simulink model "flexpwm_ctu_etimer"  (Simulink 8.1)
settings: Solver=FixedStepDiscrete  StartTime=0.0  StopTime=10.0  FixedStep=0.2  RelTol=1e-3
undefined symbols (not defined in the file or in its folder): A14, A15, B, B13, B7, D, L3, P3, PC10, PC14, PD4, PD6, R10
libraries: rappid_564xl_ec_toolbox x9
settings Model: Creator=evarshavskaya  LastModifiedBy=evarshavskaya
settings DataIOCC: ExternalInput=off  InitialState=off  SaveOutput=off  SignalLogging=off  SaveTime=off
settings OptimizationCC: InlineParams=on  OptimizeModelRefInitCode=on  LifeSpan=1
settings DebuggingCC: InheritedTsInSrcMsg=none  SingleTaskRateTransMsg=error  UnconnectedInputMsg=error  UnconnectedOutputMsg=error  UnconnectedLineMsg=error  UnknownTsInhSupMsg=error
settings HardwareCC: ProdLargestAtomicInteger=Long  ProdLargestAtomicFloat=Double  ProdIntDivRoundTo=Zero  ProdEndianess=BigEndian  ProdHWDeviceType=Freescale->32-bit PowerPC
settings RTWCC: SystemTargetFile=rappid564xl.tlc  MakeCommand=rappid_564xl_make_rtw  TemplateMakefile=rappid_564xl_default_tmf  PostCodeGenCommand=rappid_analyzegencode(buildInfo)  Description=RAppID Toolbox MPC564xL Code Generation Target (rappid)  ProcessScript=rappid564xl_make_rtw_hook
settings CodeAppCC: IgnoreCustomStorageClasses=off  CustomSymbolStrType=$N$R$M  InternalIdentifier=Classic
settings STFCustomTargetCC: CodeReplacementLibrary=ANSI_C  ModelReferenceCompliant=off  CombineOutputUpdateFcns=on  SuppressErrorStatus=on  ERTCustomFileBanners=on  SupportContinuousTime=off  SupportNonInlinedSFcns=off  MATLABClassNameForMDSCustomization=Simulink.SoftwareTarget.ERTCustomization  GRTInterface=off  SystemTargetFile=rappid564xl.tlc
settings ERTTargetCC: CodeReplacementLibrary=ANSI_C  MultiwordLength=2048  ModelReferenceCompliant=off  ParMdlRefBuildCompliant=off  CompOptLevelCompliant=off  ConcurrentExecutionCompliant=off  SuppressErrorStatus=on  ERTFirstTimeCompliant=off  ModelStepFunctionPrototypeControlCompliant=off  CPPClassGenCompliant=off  ExtModeMexFile=noextcomm  InlinedParameterPlacement=NonHierarchical  ERTCustomFileTemplate=example_file_process.tlc  ConvertIfToSwitch=off  SuppressUnreachableDefaultCases=off

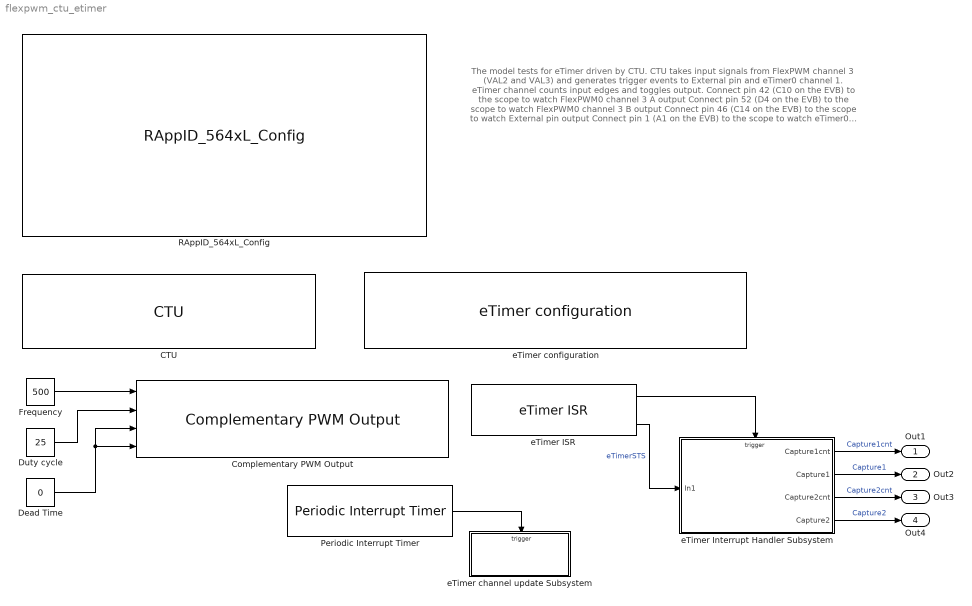
== system flexpwm_ctu_etimer ==
  note: The model tests for eTimer driven by CTU.
      |
      | CTU takes input signals from FlexPWM channel 3 (VAL2 and VAL3) and generates trigger events
      | to External pin and eTimer0 channel 1. eTimer channel counts input edges and toggles output.
      |
      | Connect pin 42 (C10 on the EVB) to the scope to watch FlexPWM0 channel 3 A output
      | Connect pin 52 (D4 on the EVB) to the scope to watch FlexPWM0 channel 3 B output
      | Connect pin 46 (C14 on the EVB) to the scope to watch External pin output
      | Connect pin 1  (A1 on the EVB) to the scope to watch eTimer0 channel 1 output
      | Connect pin 54 (D6 on the EVB) to the scope to watch eTimer0 channel 1 interrupt
  CTU : rappid_564xl_ec_toolbox/MPC564xL/Motor Control Blocks/CTU  ModeEdit=Triggered  Mode=0  MRSedit=PWM reload Rising edge  MRS=0  MaxDelay=1000  ExtTgrPin_0="46  : PC14 : [ 103 ] : [ E15 ]"  ExtInPin_0=None  extTgrPcr=46  extInPcr=255  InputSelection=16843008  PWM_REL=Disabled  PWM_ODD_0=Disabled  PWM_ODD_1=Disabled  PWM_ODD_2=Disabled  PWM_ODD_3=Rising  PWM_EVEN_0=Disabled  PWM_EVEN_1=Disabled  PWM_EVEN_2=Disabled  PWM_EVEN_3=Rising  RPWM_0=Disabled  RPWM_1=Disabled  RPWM_2=Disabled  RPWM_3=Rising  eTimer_0=Disabled  eTimer_1=Disabled  External=Disabled  TriggerOutput_1=98  TriggerOutput_2=0  ADC_CmdIndex_1=0  ADC_CmdIndex_2=0  ADC_Cmd_1=16384  ADC_Cmd_2=0  ADC_Cmd_3=0  ADC_Cmd_4=0  ADC_Cmd_5=0  ADC_Cmd_6=0  ADC_Cmd_7=0  ADC_Cmd_8=0  ADC_Cmd_9=0  ADC_Cmd_10=0  ADC_Cmd_11=0  ADC_Cmd_12=0  ADC_Cmd_13=0  ADC_Cmd_14=0  ADC_Cmd_15=0  ADC_Cmd_16=0  ADC_Cmd_17=0  ADC_Cmd_18=0  ADC_Cmd_19=0  ADC_Cmd_20=0  ADC_Cmd_21=0  ADC_Cmd_22=0  ADC_Cmd_23=0  ADC_Cmd_24=0  T0_E=on  T0_ETE=on  T0_T0E=on  T0_T1E=off  T0_T2E=off  T0_ADCE=off  T0_Delay=250  T1_E=off  T1_ETE=off  T1_T0E=off  T1_T1E=off  T1_T2E=off  T1_ADCE=off  T1_Delay=250  T2_E=off  T2_ETE=off  T2_T0E=off  T2_T1E=off  T2_T2E=off  T2_ADCE=off  T2_Delay=0  T3_E=off  T3_ETE=off  T3_T0E=off  T3_T1E=off  T3_T2E=off  T3_ADCE=off  T3_Delay=0  T4_E=off  T4_ETE=off  T4_T0E=off  T4_T1E=off  T4_T2E=off  T4_ADCE=off  T4_Delay=0  T5_E=off  T5_ETE=off  T5_T0E=off  T5_T1E=off  T5_T2E=off  T5_ADCE=off  T5_Delay=0  T6_E=off  T6_ETE=off  T6_T0E=off  T6_T1E=off  T6_T2E=off  T6_ADCE=off  T6_Delay=0  T7_E=off  T7_ETE=off  T7_T0E=off  T7_T1E=off  T7_T2E=off  T7_ADCE=off  T7_Delay=0  T_delay=0  ADC_Cmd=0  T0_ADC_num=0  T0_ADC_nlist=no commands  T1_ADC_num=0  T1_ADC_nlist=no commands  T2_ADC_num=0  T2_ADC_nlist=no commands  T3_ADC_num=0  T3_ADC_nlist=no commands  T4_ADC_num=0  T4_ADC_nlist=no commands  T5_ADC_num=0  T5_ADC_nlist=no commands  T6_ADC_num=0  T6_ADC_nlist=no commands  T7_ADC_num=0  T7_ADC_nlist=no commands  ADC_CMS_1=Single-conversion mode: ADC unit A  ADC_CIR_1=Disabled  ADC_FIFO_1=0  ADC_CHA_1=0  ADC_CHB_1=0  ADC_CMS_2=Single-conversion mode: ADC unit A  ADC_CIR_2=Disabled  ADC_FIFO_2=0  ADC_CHA_2=0  ADC_CHB_2=0  ADC_CMS_3=Single-conversion mode: ADC unit A  ADC_CIR_3=Disabled  ADC_FIFO_3=0  ADC_CHA_3=0  ADC_CHB_3=0  ADC_CMS_4=Single-conversion mode: ADC unit A  ADC_CIR_4=Disabled  ADC_FIFO_4=0  ADC_CHA_4=0  ADC_CHB_4=0  ADC_CMS_5=Single-conversion mode: ADC unit A  ADC_CIR_5=Disabled  ADC_FIFO_5=0  ADC_CHA_5=0  ADC_CHB_5=0  ADC_CMS_6=Single-conversion mode: ADC unit A  ADC_CIR_6=Disabled  ADC_FIFO_6=0  ADC_CHA_6=0  ADC_CHB_6=0  ADC_CMS_7=Single-conversion mode: ADC unit A  ADC_CIR_7=Disabled  ADC_FIFO_7=0  ADC_CHA_7=0  ADC_CHB_7=0  ADC_CMS_8=Single-conversion mode: ADC unit A  ADC_CIR_8=Disabled  ADC_FIFO_8=0  ADC_CHA_8=0  ADC_CHB_8=0  ADC_CMS_9=Single-conversion mode: ADC unit A  ADC_CIR_9=Disabled  ADC_FIFO_9=0  ADC_CHA_9=0  ADC_CHB_9=0  ADC_CMS_10=Single-conversion mode: ADC unit A  ADC_CIR_10=Disabled  ADC_FIFO_10=0  ADC_CHA_10=0  ADC_CHB_10=0  ADC_CMS_11=Single-conversion mode: ADC unit A  ADC_CIR_11=Disabled  ADC_FIFO_11=0  ADC_CHA_11=0  ADC_CHB_11=0  ADC_CMS_12=Single-conversion mode: ADC unit A  ADC_CIR_12=Disabled  ADC_FIFO_12=0  ADC_CHA_12=0  ADC_CHB_12=0  ADC_CMS_13=Single-conversion mode: ADC unit A  ADC_CIR_13=Disabled  ADC_FIFO_13=0  ADC_CHA_13=0  ADC_CHB_13=0  ADC_CMS_14=Single-conversion mode: ADC unit A  ADC_CIR_14=Disabled  ADC_FIFO_14=0  ADC_CHA_14=0  ADC_CHB_14=0  ADC_CMS_15=Single-conversion mode: ADC unit A  ADC_CIR_15=Disabled  ADC_FIFO_15=0  ADC_CHA_15=0  ADC_CHB_15=0  ADC_CMS_16=Single-conversion mode: ADC unit A  ADC_CIR_16=Disabled  ADC_FIFO_16=0  ADC_CHA_16=0  ADC_CHB_16=0  ADC_CMS_17=Single-conversion mode: ADC unit A  ADC_CIR_17=Disabled  ADC_FIFO_17=0  ADC_CHA_17=0  ADC_CHB_17=0  ADC_CMS_18=Single-conversion mode: ADC unit A  ADC_CIR_18=Disabled  ADC_FIFO_18=0  ADC_CHA_18=0  ADC_CHB_18=0  ADC_CMS_19=Single-conversion mode: ADC unit A  ADC_CIR_19=Disabled  ADC_FIFO_19=0  ADC_CHA_19=0  ADC_CHB_19=0  ADC_CMS_20=Single-conversion mode: ADC unit A  ADC_CIR_20=Disabled  ADC_FIFO_20=0  ADC_CHA_20=0  ADC_CHB_20=0  ADC_CMS_21=Single-conversion mode: ADC unit A  ADC_CIR_21=Disabled  ADC_FIFO_21=0  ADC_CHA_21=0  ADC_CHB_21=0  ADC_CMS_22=Single-conversion mode: ADC unit A  ADC_CIR_22=Disabled  ADC_FIFO_22=0  ADC_CHA_22=0  ADC_CHB_22=0  ADC_CMS_23=Single-conversion mode: ADC unit A  ADC_CIR_23=Disabled  ADC_FIFO_23=0  ADC_CHA_23=0  ADC_CHB_23=0  ADC_CMS_24=Single-conversion mode: ADC unit A  ADC_CIR_24=Disabled  ADC_FIFO_24=0  ADC_CHA_24=0  ADC_CHB_24=0  dst=|  T0_cmdNum=1  T0_ADC_CMS_1=Single-conversion mode: ADC unit A  T0_ADC_CIR_1=Disabled  T0_ADC_FIFO_1=0  T0_ADC_CHA_1=0  T0_ADC_CHB_1=0  T0_ADC_CMS_2=Single-conversion mode: ADC unit A  T0_ADC_CIR_2=Disabled  T0_ADC_FIFO_2=0  T0_ADC_CHA_2=0  T0_ADC_CHB_2=0  T0_ADC_CMS_3=Single-conversion mode: ADC unit A  T0_ADC_CIR_3=Disabled  T0_ADC_FIFO_3=0  T0_ADC_CHA_3=0  T0_ADC_CHB_3=0  T1_cmdNum=1  T1_ADC_CMS_1=Single-conversion mode: ADC unit A  T1_ADC_CIR_1=Disabled  T1_ADC_FIFO_1=0  T1_ADC_CHA_1=3  T1_ADC_CHB_1=0  T1_ADC_CMS_2=Single-conversion mode: ADC unit A  T1_ADC_CIR_2=Disabled  T1_ADC_FIFO_2=0  T1_ADC_CHA_2=0  T1_ADC_CHB_2=0  T1_ADC_CMS_3=Single-conversion mode: ADC unit A  T1_ADC_CIR_3=Disabled  T1_ADC_FIFO_3=0  T1_ADC_CHA_3=0  T1_ADC_CHB_3=0  ver=2
      | Triggered mode
      |       Input selection: 00000001 00000001 00000001 00000000
      | Trigger Output 0-3: 00000000 00000000 00000000 01100010
      | Trigger Output 4-7: 00000000 00000000 00000000 00000000
      | ADC command list size: 0
  Complementary PWM Output : rappid_564xl_ec_toolbox/MPC564xL/Motor Control Blocks/Complementary PWM Output  pwmModule=0  pwmMod=0  SubModule=3  subMod=3  InitFreq=500  resolution=1 %  resValue=1  InitDuty=25  pwm45=off  pwm45en=0  InitDutyB=0  DeadTime=0  dt=IPBus clock cycles  deadtime_mks=0  debugSw=off  debug_mode=0  pin_A0=None  pin_B0=None  pin_A1=None  pin_B1=None  pin_A2=None  pin_B2=None  pin_A3="42  : PC10 : [ 111 ] : [ A15 ]"  pin_B3="52  : PD4  : [ 129 ] : [ B7 ]"  pin1_A0=None  pin1_B0=None  pin1_A1=None  pin1_B1=None  pin1_A2=None  pin1_B2=None  pin1_A3=None  pin1_B3=None  pcrNumA=42  pcrNumB=52  polA=off  polB=off  octrl=0  syncFrom0=off  masterSync=0  outVal0=off  outVal1=off  outVal2=on  outVal3=on  outVal4=on  outVal5=on  outTrig=12
  Dead Time : Constant  Value=0  OutDataTypeStr=uint32
  Duty cycle : Constant  Value=25  OutDataTypeStr=uint32
  Frequency : Constant  Value=500  OutDataTypeStr=uint32
  Periodic Interrupt Timer : rappid_564xl_ec_toolbox/MPC564xL/General Purpose Blocks/Periodic Interrupt Timer  pit_chan=1  pit_timeout=200  int_priority=13  pit_timeout_val=23999999
  RAppID_564xL_Config : rappid_564xl_ec_toolbox/MPC564xL/RAppID_564xL_Config  SystemClock=120  XTAL=40  MC_clock_60=12  MC_clock_80=16  MC_clock_120=10  SWG_clock_60=20  SWG_clock_80=13.334  SWG_clock_120=20  Compiler=CodeWarrior  MemTarget=RAM  Part=MPC5643L  Package=144 LQFP  global_int_priority=10  base_tick_priority=14  sys_task_supress=off  exception_handlers=off  stored_mdl_name=flexpwm_ctu_etimer  freemaster_interface=Oops  freemaster_rx_pin="LINFlex_0 Rx Pin 116 : \"PB[3]\""  freemaster_tx_pin="LINFlex_0 Tx Pin 114 : \"PB[2]\""  freemaster_interface_1=None  freemaster_enable=off  freemaster_rate=57600  freemaster_tx0_pin=18 : B[2] : 114 : A14  freemaster_rx0_pin=19 : B[3] : 116 : B13  freemaster_tx1_pin=57 : D[9] : 26 : L3  freemaster_rx1_pin=29 : B[13] : 60 : R10  freemaster_can_channel=1CH  freemater_can_speed=500K  freemaster_can_msgig=0x7AA  ccp_interface=None  ccp_enable=off  ccp_can_channel=CH1 (MB 0 - 1)  ccp_can_speed=500K  ccp_can_cro_id=256  ccp_can_dto_id=257  ccp_dev_id=RappID  ccp_dev_addr=0  ccp_odt=3  ccp_daq=3  pil_enable=off  pil_bam=on  comport=1  pil_rate=57600  bam_password_def=on  bam_password=0xFEEDFACECAFEBEEF  bam_sa_cs=off  bam_start_address=0x0  bam_code_size=0x7000  cons_dspi=on  cons_can=on  cons_adc=on  cons_pwm=on  cons_ctu=on  cons_swg=on  cons_eTimer=on  cons_fm=on
  eTimer ISR : rappid_564xl_ec_toolbox/MPC564xL/Motor Control Blocks/eTimer ISR  SubModule=0  Timerchan=1  subMod=0  channel=1  isrPriority=12  isrPrio=12
  eTimer Interrupt Handler Subsystem : Subsystem  TreatAsAtomicUnit=on
      settings: RTWSystemCode=Nonreusable function
  eTimer channel update Subsystem : Subsystem  TreatAsAtomicUnit=on
      settings: RTWSystemCode=Nonreusable function
  eTimer configuration : rappid_564xl_ec_toolbox/MPC564xL/Motor Control Blocks/eTimer configuration  SubModule=0  TimerChan=1  subMod=0  channel=1  CountMode=010 - Count rising and falling edges of primary source  CNTMODE=2  CountOnce=0 - Count repeatedly  ONCE=0  CountLength=1 - Count until compare and then reinitialize  LENGTH=1  CountDirection=0 - Count up  DIR=0  OutputEnable=1 - Output signal is driven to the external pin  OEN=1  CoChanInit=00 - Other channels cannot force re-initialization of this channel  COINIT=0  StopAction=0 - Output enable is unaffected by stop mode  STPEN=0  ReloadOnCapt=00 - Do not reload the counter on a capture event  ROC=0  PrimarySource=01000 - Auxiliary input #0 pin  PRISRC=8  PrimSrcPol=0 - True polarity  PIPS=0  SecondarySource=01000 - Auxiliary input #0 pin  SECSRC=8  SecSrcPol=0 - True polarity  SIPS=0  FILT_CNT=0  FILT_PER=0  FILT=0  OutputMode=0011 - Toggle output on successful compare (COMP1 or COMP2)  OUTMODE=3  OutputPol=0 - True polarity  OPS=0  MasterMode=0 - Disable broadcast of this channel output  MSTR=0  ForcedOutVal=0  VAL=0  CoForce=0 - Other channels cannot force this channel output  COFRC=0  CompLoad1=010 - Load COMP1 with CMPLD1 upon successful compare with the value in COMP1  CLC1=2  CompLoad2=101 - Load COMP2 with CMPLD2 upon successful compare with the value in COMP2  CLC2=5  CompareMode="00 - COMP1 and COMP2  are used when the counter is counting up"  CMPMODE=0  CaptMode1=10 - Capture rising edges  CPT1MODE=2  CaptMode2=00 - Capture disabled  CPT2MODE=0  OneShCaptMode=0 - Free running mode is selected  ONESHOT=0  CaptFIFO=0  CFWM=0  CNTRinit=1  COMP1init=10  COMP2init=20  mod0ch0pin=None  mod0ch1pin="1   : PA1  : [ 74 ] : [ R14 ]  input/output"  mod0ch2pin=None  mod0ch3pin=None  mod0ch4pin=None  mod0ch5pin=None  mod1ch0pin=None  mod1ch1pin=None  mod1ch2pin=None  mod1ch3pin=None  mod1ch4pin=None  mod1ch5pin=None  mod2ch0pin=None  mod2ch1pin=None  mod2ch2pin=None  mod2ch3pin=None  mod2ch4pin=None  mod2ch5pin=None  pcrNum0=255  pcrNum1=1  pcrNum2=255  pcrNum3=255  pcrNum4=255  pcrNum5=255  TCFIE=off  TCF1IE=off  TCF2IE=off  TOFIE=off  IELFIE=off  IEHFIE=off  ICF1IE=on  ICF2IE=off  INTDMA=64
  Out1 : Outport
  Out2 : Outport  Port=2
  Out3 : Outport  Port=3
  Out4 : Outport  Port=4
  wires:
  Frequency/1 -> Complementary PWM Output/1
  Duty cycle/1 -> Complementary PWM Output/2
  Dead Time/1 -> Complementary PWM Output/3, Complementary PWM Output/4
  eTimer ISR/1 -> eTimer Interrupt Handler Subsystem/Trigger
  Periodic Interrupt Timer/1 -> eTimer channel update Subsystem/Trigger
  eTimer Interrupt Handler Subsystem/1(Capture1cnt) -> Out1/1  "Capture1cnt"
  eTimer Interrupt Handler Subsystem/2(Capture1) -> Out2/1  "Capture1"
  eTimer Interrupt Handler Subsystem/3(Capture2cnt) -> Out3/1  "Capture2cnt"
  eTimer Interrupt Handler Subsystem/4(Capture2) -> Out4/1  "Capture2"
  eTimer ISR/2 -> eTimer Interrupt Handler Subsystem/1(In1)  "eTimerSTS"

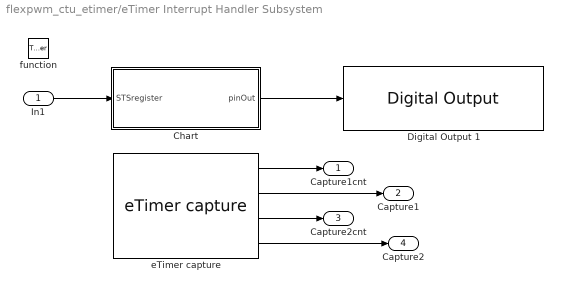
== system flexpwm_ctu_etimer/eTimer Interrupt Handler Subsystem ==
  In1 : Inport
  function : TriggerPort  TriggerType=function-call
  Chart : Stateflow chart  TreatAsAtomicUnit=on
  Digital Output 1 : rappid_564xl_ec_toolbox/MPC564xL/General Purpose Blocks/Digital Output   gpio_outputs="54  : PD6  : [ 34 ] : [ P3 ]"  pinNum=[ 34 ]  pcrNum=54
  eTimer capture : rappid_564xl_ec_toolbox/MPC564xL/Motor Control Blocks/eTimer capture  SubModule=0  Timerchan=1  subMod=0  channel=1
  Capture1cnt : Outport
  Capture1 : Outport  Port=2
  Capture2cnt : Outport  Port=3
  Capture2 : Outport  Port=4
  wires:
  eTimer capture/1 -> Capture1cnt/1
  eTimer capture/2 -> Capture1/1
  In1/1 -> Chart/1(STSregister)
  Chart/1(pinOut) -> Digital Output 1/1
  eTimer capture/3 -> Capture2cnt/1
  eTimer capture/4 -> Capture2/1

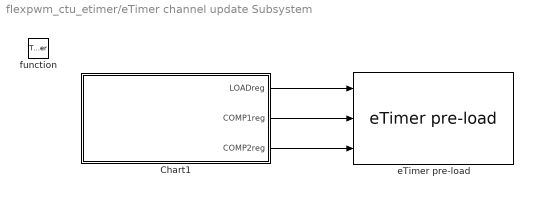
== system flexpwm_ctu_etimer/eTimer channel update Subsystem ==
  function : TriggerPort  TriggerType=function-call
  Chart1 : Stateflow chart  TreatAsAtomicUnit=on
  eTimer pre-load : rappid_564xl_ec_toolbox/MPC564xL/Motor Control Blocks/eTimer pre-load  SubModule=0  Timerchan=1  subMod=0  channel=1
  wires:
  Chart1/1(LOADreg) -> eTimer pre-load/1
  Chart1/2(COMP1reg) -> eTimer pre-load/2
  Chart1/3(COMP2reg) -> eTimer pre-load/3

== stateflow chart eTimer channel update Subsystem/Chart1 ==
  settings: executeAtInitialization=1
  state A
    du:
    LOADreg=1;
    COMP1reg=20;
    COMP2reg=20;
    int_counter=int_counter+1;
  state A1
    du:
    LOADreg=1;
    COMP1reg=10;
    COMP2reg=10;
    int_counter=int_counter-1;
  (default) -> A : {int_counter=0;}
  A1 -> A : [int_counter < 2]
  A -> A1 : [int_counter > 10]
  data: LOADreg output uint16 [0..100]; COMP1reg output uint16 [0..100]; int_counter local uint32 [0..1000] =0; COMP2reg output uint16 [0..100]

== stateflow chart eTimer Interrupt Handler Subsystem/Chart ==
  state A
    du:
    compare = STSregister & 2;
    en:
    compare = STSregister & 2;
    pinOut = 1;
  state A1
    du:
    compare = STSregister & 2;
    en:
    compare = STSregister & 2;
    pinOut = 0;
  (default) -> A
  A -> A1 : [compare == 0]
  A1 -> A : [compare != 0]
  data: compare local int16 [0..2]; pinOut output boolean [0..1]; STSregister input uint16 [0..65535]
